simulink model "Simplified_UAV_Task3"  (R2024b)
settings: Solver=VariableStepAuto  StartTime=0  StopTime=3000  FixedStep=1e-4  RelTol=1e-5  AbsTol=1e-5
values from neighbouring files (symbols this model uses):
  adaptiveActivation = 1    [Simplified_UAV_Task3_main.m]    (also in newUAV_Task3_main.m)
  B_p = 1/UAV.m    [Simplified_UAV_Task3_main.m]    (also in newUAV_Task3_main.m)
  Gamma_a = 1*[1 1 1 1]'    [Simplified_UAV_Task3_main.m]    (also in newUAV_Task3_main.m = 2*[1 1 1 1]')
  gravityInAdaptiveController = 1    [Simplified_UAV_Task3_main.m]    (also in newUAV_Task3_main.m)
  L = 10    [Simplified_UAV_Task3_main.m]    (also in newUAV_Task3_main.m)
  lambda = 0.89    [Simplified_UAV_Task3_main.m]    (also in newUAV_Task3_main.m)
  lambda_0 = 1    [Simplified_UAV_Task3_main.m]    (also in newUAV_Task3_main.m)
  p_0 = [0; 0; 0]    [Simplified_UAV_Task3_main.m]    (also in newUAV_Task3_main.m)
  PO = 1    [Simplified_UAV_Task3_main.m]    (also in newUAV_Task3_main.m)
  scenario = 2    [Simplified_UAV_Task3_main.m]    (also in newUAV_Task3_main.m)
  theta_0 = [0.07;0.07;0.1]    [Simplified_UAV_Task3_main.m]    (also in newUAV_Task3_main.m)
  vb_0 = [0; 0; 0]    [Simplified_UAV_Task3_main.m]    (also in newUAV_Task3_main.m)
undefined symbols (not defined in the file or in its folder): ctrl, epsilon_PO, g, Gamma_a_scalar, par, projection_operator, targetParams, theta_M, UAV, v_0
libraries: matrix_library x12, slpidlib x12, spsRMSLib x1, uavutilslib x1
(part 3 of 3)

== system Simplified_UAV_Task3/Position Controller/ADAPTIVE CONTROLLER/Subsystem1 ==
  u_b : Inport
  lambda : Inport  Port=2
  xp : Inport  Port=3
  thetap_hat : Inport  Port=4
  Constant : Constant
  Create Diagonal Matrix : matrix_library/Create Diagonal Matrix
  Gain2 : Gain  Gain=-1
  MATLAB Function1 : MATLAB Function  TreatAsAtomicUnit=on
  Matrix Multiply : Product
  Matrix Multiply1 : Product  Multiplication=Matrix(*)
  Matrix Multiply2 : Product
  Sum : Sum  Inputs=+-
  Sum1 : Sum  Inputs=+-
  Sum2 : Sum
  u_a : Outport
  u : Outport  Port=2
  wires:
  lambda/1 -> MATLAB Function1/1(lambda)
  MATLAB Function1/1(Lambda_hat_inv) -> Matrix Multiply2/1, Sum/1
  Constant/1 -> Sum/2
  Sum/1 -> Matrix Multiply/1
  u_b/1 -> Sum2/2, Matrix Multiply/2
  Matrix Multiply/1 -> Sum1/1
  xp/1 -> Create Diagonal Matrix/1
  thetap_hat/1 -> Matrix Multiply1/2
  Sum1/1 -> Sum2/1, u_a/1
  Sum2/1 -> u/1
  Create Diagonal Matrix/1 -> Gain2/1
  Gain2/1 -> Matrix Multiply1/1
  Matrix Multiply1/1 -> Matrix Multiply2/2
  Matrix Multiply2/1 -> Sum1/2

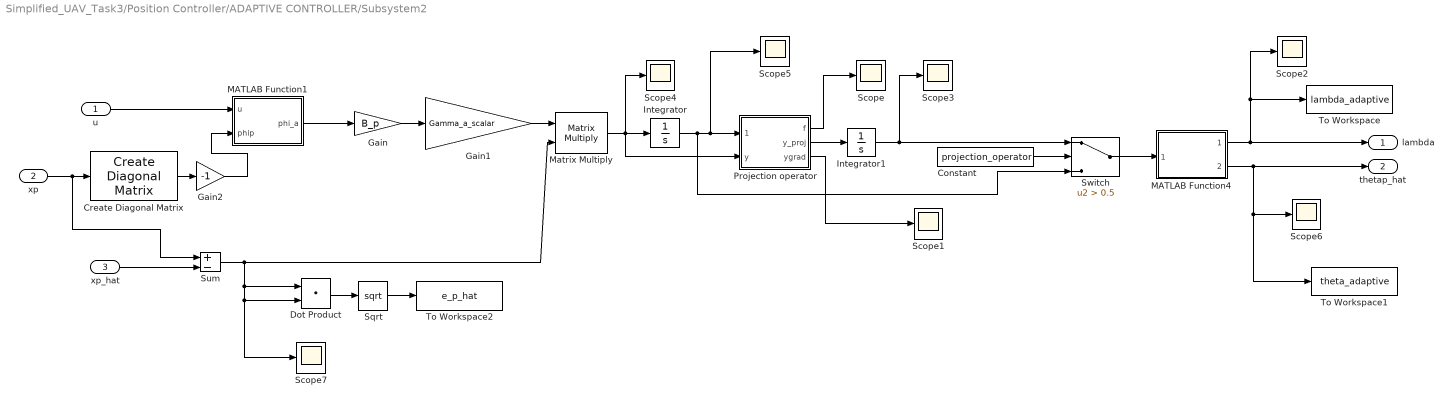
== system Simplified_UAV_Task3/Position Controller/ADAPTIVE CONTROLLER/Subsystem2 ==
  u : Inport
  xp : Inport  Port=2
  xp_hat : Inport  Port=3
  Constant : Constant  Value=projection_operator
  Create Diagonal Matrix : matrix_library/Create Diagonal Matrix
  Dot Product : DotProduct  OutDataTypeStr=Inherit: Inherit via internal rule
  Gain : Gain  Gain=B_p
  Gain1 : Gain  Gain=Gamma_a_scalar
  Gain2 : Gain  Gain=-1
  Integrator : Integrator  InitialCondition=[lambda_0; theta_0]
  Integrator1 : Integrator  InitialCondition=[lambda_0; theta_0]
  MATLAB Function1 : MATLAB Function  TreatAsAtomicUnit=on
  MATLAB Function4 : MATLAB Function  TreatAsAtomicUnit=on
  Matrix Multiply : Product  Multiplication=Matrix(*)
  Projection operator : MATLAB Function  TreatAsAtomicUnit=on
  Scope{,1..7} (8 alike) : Scope
  Sqrt : Sqrt
  Sum : Sum  Inputs=+-
  Switch : Switch  Criteria=u2 > Threshold  Threshold=0.5  SaturateOnIntegerOverflow=off  InputSameDT=off
  To Workspace : ToWorkspace  VariableName=lambda_adaptive  SaveFormat=Timeseries  SampleTime=-1
  To Workspace1 : ToWorkspace  VariableName=theta_adaptive  SaveFormat=Timeseries  SampleTime=-1
  To Workspace2 : ToWorkspace  VariableName=e_p_hat  SaveFormat=Timeseries  SampleTime=-1
  lambda : Outport
  thetap_hat : Outport  Port=2
  wires:
  u/1 -> MATLAB Function1/1(u)
  xp_hat/1 -> Sum/2
  MATLAB Function1/1(phi_a) -> Gain/1
  Gain/1 -> Gain1/1
  Gain1/1 -> Matrix Multiply/1
  Matrix Multiply/1 -> Projection operator/2(y), Scope4/1, Integrator/1
  Integrator/1 -> Switch/3, Scope5/1, Projection operator/1(theta_a_hat)
  Projection operator/3(ygrad) -> Scope1/1
  Projection operator/1(f) -> Scope/1
  MATLAB Function4/2(thetap_hat) -> To Workspace1/1, Scope6/1, thetap_hat/1
  Integrator1/1 -> Switch/1, Scope3/1
  Projection operator/2(y_proj) -> Integrator1/1
  xp/1 -> Create Diagonal Matrix/1, Sum/1
  Switch/1 -> MATLAB Function4/1(theta_a)
  Constant/1 -> Switch/2
  Create Diagonal Matrix/1 -> Gain2/1
  Gain2/1 -> MATLAB Function1/2(phip)
  Sqrt/1 -> To Workspace2/1
  Sum/1 -> Scope7/1, Dot Product/2, Dot Product/1, Matrix Multiply/2
  Dot Product/1 -> Sqrt/1
  MATLAB Function4/1(lambda) -> lambda/1, To Workspace/1, Scope2/1

== system Simplified_UAV_Task3/Position Controller/Adaptive Augmentation/Predictor (x_p_hat) dynamics ==
  Lambda_hat : Inport
  u : Inport  Port=2
  phi_p : Inport  Port=3
  theta_p_hat : Inport  Port=4
  x_p : Inport  Port=5
  Add : Sum
  Constant : Constant  Value=g*e3
  Gain : Gain  Gain=B_p  Multiplication=Matrix(K*u)
  Gain1 : Gain  Gain=L
  Gain2 : Gain  Gain=gravityInAdaptiveController
  Gain3 : Gain
  Integrator : Integrator  InitialCondition=v_0
  Matrix Multiply : Product
  Matrix Multiply1 : Product  Multiplication=Matrix(*)
  Reshape : Reshape  OutputDimensionality=Column vector (2-D)
  Reshape1 : Reshape  OutputDimensionality=Column vector (2-D)
  Reshape2 : Reshape  OutputDimensionality=Column vector (2-D)
  Scope : Scope
  Scope1 : Scope
  Sum : Sum  Inputs=+++
  Sum1 : Sum  Inputs=-+|
  Transpose : Math  Operator=transpose
  x_p_hat : Outport
  wires:
  Lambda_hat/1 -> Matrix Multiply/1
  Matrix Multiply/1 -> Add/1
  phi_p/1 -> Transpose/1
  theta_p_hat/1 -> Matrix Multiply1/2
  Matrix Multiply1/1 -> Add/2
  Add/1 -> Gain/1
  Gain/1 -> Reshape1/1
  Gain1/1 -> Reshape/1
  x_p/1 -> Scope1/1, Sum1/2
  Sum1/1 -> Gain1/1
  Integrator/1 -> Scope/1, Sum1/1, x_p_hat/1
  Sum/1 -> Integrator/1
  Reshape/1 -> Sum/1
  Reshape1/1 -> Sum/2
  Reshape2/1 -> Sum/3
  Constant/1 -> Gain2/1
  Transpose/1 -> Matrix Multiply1/1
  u/1 -> Matrix Multiply/2
  Gain2/1 -> Gain3/1
  Gain3/1 -> Reshape2/1

== system Simplified_UAV_Task3/Position Controller/Adaptive Augmentation/Subsystem ==
  Lambda_hat : Inport
  u_b : Inport  Port=2
  phi_p : Inport  Port=3
  theta_p_hat : Inport  Port=4
  Constant : Constant  Value=eye(3,3)
  Gain : Gain  Commented=through  Gain=-1
  Gain1 : Gain
  Inverse : MATLAB Function  TreatAsAtomicUnit=on
  Product : Product  Multiplication=Matrix(*)
  Product1 : Product  Inputs=3  Multiplication=Matrix(*)
  Subtract : Sum  Inputs=-+
  Subtract1 : Sum  Inputs=+-
  Transpose : Math  Operator=transpose
  u_a : Outport
  wires:
  Lambda_hat/1 -> Inverse/1(u)
  Inverse/1(y) -> Product1/1, Subtract/2
  Constant/1 -> Subtract/1
  Subtract/1 -> Product/1
  u_b/1 -> Product/2
  Product/1 -> Gain1/1
  Subtract1/1 -> u_a/1
  phi_p/1 -> Transpose/1
  Transpose/1 -> Gain/1
  theta_p_hat/1 -> Product1/3
  Product1/1 -> Subtract1/2
  Gain/1 -> Product1/2
  Gain1/1 -> Subtract1/1

== system Simplified_UAV_Task3/Position Controller/Adaptive Augmentation/phi_a ==
  u : Inport
  phi_p : Inport  Port=2
  Matrix Concatenate : Concatenate  Mode=Multidimensional array
  Scope : Scope
  Transpose : Math  Operator=transpose
  phi_a : Outport
  wires:
  Matrix Concatenate/1 -> Scope/1, phi_a/1
  u/1 -> Transpose/1
  phi_p/1 -> Matrix Concatenate/2
  Transpose/1 -> Matrix Concatenate/1

== system Simplified_UAV_Task3/Position Controller/Adaptive Augmentation/phi_p ==
  x_p : Inport
  Create Diagonal Matrix : matrix_library/Create Diagonal Matrix
  Gain : Gain  Gain=-1
  phi_p : Outport
  wires:
  x_p/1 -> Gain/1
  Gain/1 -> Create Diagonal Matrix/1
  Create Diagonal Matrix/1 -> phi_p/1

== system Simplified_UAV_Task3/Position Controller/Adaptive Augmentation/theta_a_hat dynamics ==
  Gamma_a : Inport
  phi_a : Inport  Port=2
  B_p : Inport  Port=3
  x_p : Inport  Port=4
  x_p_hat : Inport  Port=5
  Constant1 : Constant  Value=PO
  Dot Product : DotProduct  OutDataTypeStr=Inherit: Inherit via internal rule
  Integrator : Integrator  InitialCondition=[lambda_0; theta_0]
  Matrix Multiply1 : Product
  Matrix Multiply2 : Product  Multiplication=Matrix(*)
  Matrix Multiply3 : Product
  Projection operator : Subsystem
  Scope{,1..4} (5 alike) : Scope
  Sqrt : Sqrt
  Subtract : Sum  Inputs=+-
  Switch : Switch  Criteria=u2 > Threshold  SaturateOnIntegerOverflow=off  InputSameDT=off
  To Workspace : ToWorkspace  VariableName=e_p_hat  SaveFormat=Timeseries  SampleTime=-1
  Transpose : Math  Operator=transpose
  Transpose1 : Math  Commented=through  Operator=transpose
  theta_a_hat : Outport
  wires:
  x_p_hat/1 -> Subtract/2
  B_p/1 -> Transpose/1
  Subtract/1 -> Scope4/1, Dot Product/2, Dot Product/1, Matrix Multiply1/2
  Transpose/1 -> Matrix Multiply1/1
  phi_a/1 -> Transpose1/1
  Matrix Multiply1/1 -> Scope3/1, Matrix Multiply2/2
  Gamma_a/1 -> Matrix Multiply3/1
  Matrix Multiply2/1 -> Matrix Multiply3/2
  Matrix Multiply3/1 -> Projection operator/1(theta_dot), Scope2/1, Integrator/1
  x_p/1 -> Subtract/1
  Constant1/1 -> Switch/2, Projection operator/Enable
  Integrator/1 -> Scope1/1, Switch/3
  Switch/1 -> theta_a_hat/1
  Projection operator/1(theta) -> Scope/1, Switch/1
  Dot Product/1 -> Sqrt/1
  Sqrt/1 -> To Workspace/1
  Transpose1/1 -> Matrix Multiply2/1

== system Simplified_UAV_Task3/Position Controller/Adaptive Augmentation to delete/Predictor (x_p_hat) dynamics ==
  Lambda_hat : Inport
  u : Inport  Port=2
  phi_p : Inport  Port=3
  theta_p_hat : Inport  Port=4
  x_p : Inport  Port=5
  Add : Sum
  Constant : Constant  Value=g*e3
  Gain : Gain  Gain=B_p  Multiplication=Matrix(K*u)
  Gain1 : Gain  Gain=L
  Integrator : Integrator  InitialCondition=v_0
  Matrix Multiply : Product
  Matrix Multiply1 : Product  Multiplication=Matrix(*)
  Reshape : Reshape  OutputDimensionality=Column vector (2-D)
  Reshape1 : Reshape  OutputDimensionality=Column vector (2-D)
  Reshape2 : Reshape  OutputDimensionality=Column vector (2-D)
  Scope : Scope
  Sum : Sum  Inputs=+++
  Sum1 : Sum  Inputs=-+|
  Transpose : Math  Operator=transpose
  x_p_hat : Outport
  wires:
  Lambda_hat/1 -> Matrix Multiply/1
  u/1 -> Matrix Multiply/2
  Matrix Multiply/1 -> Add/1
  phi_p/1 -> Transpose/1
  theta_p_hat/1 -> Matrix Multiply1/2
  Matrix Multiply1/1 -> Add/2
  Add/1 -> Gain/1
  Gain/1 -> Reshape1/1
  Gain1/1 -> Reshape/1
  x_p/1 -> Sum1/2
  Sum1/1 -> Gain1/1
  Integrator/1 -> Scope/1, Sum1/1, x_p_hat/1
  Sum/1 -> Integrator/1
  Reshape/1 -> Sum/1
  Reshape1/1 -> Sum/2
  Reshape2/1 -> Sum/3
  Constant/1 -> Reshape2/1
  Transpose/1 -> Matrix Multiply1/1

== system Simplified_UAV_Task3/Position Controller/Adaptive Augmentation to delete/Subsystem ==
  Lambda_hat : Inport
  u_b : Inport  Port=2
  phi_p : Inport  Port=3
  theta_p_hat : Inport  Port=4
  Constant : Constant  Value=eye(3,3)
  Gain : Gain  Commented=through  Gain=-1
  Gain1 : Gain
  Inverse : MATLAB Function  TreatAsAtomicUnit=on
  Product : Product  Multiplication=Matrix(*)
  Product1 : Product  Inputs=3  Multiplication=Matrix(*)
  Subtract : Sum  Inputs=-+
  Subtract1 : Sum  Inputs=+-
  Transpose : Math  Operator=transpose
  u_a : Outport
  wires:
  Lambda_hat/1 -> Inverse/1(u)
  Inverse/1(y) -> Product1/1, Subtract/2
  Constant/1 -> Subtract/1
  Subtract/1 -> Product/1
  u_b/1 -> Product/2
  Product/1 -> Gain1/1
  Subtract1/1 -> u_a/1
  phi_p/1 -> Transpose/1
  Transpose/1 -> Gain/1
  theta_p_hat/1 -> Product1/3
  Product1/1 -> Subtract1/2
  Gain/1 -> Product1/2
  Gain1/1 -> Subtract1/1

== system Simplified_UAV_Task3/Position Controller/Adaptive Augmentation to delete/phi_a ==
  u : Inport
  phi_p : Inport  Port=2
  Matrix Concatenate : Concatenate  Mode=Multidimensional array
  Scope : Scope
  Transpose : Math  Operator=transpose
  phi_a : Outport
  wires:
  Matrix Concatenate/1 -> Scope/1, phi_a/1
  u/1 -> Transpose/1
  phi_p/1 -> Matrix Concatenate/2
  Transpose/1 -> Matrix Concatenate/1

== system Simplified_UAV_Task3/Position Controller/Adaptive Augmentation to delete/phi_p ==
  x_p : Inport
  Create Diagonal Matrix : matrix_library/Create Diagonal Matrix
  Gain : Gain  Gain=-1
  phi_p : Outport
  wires:
  x_p/1 -> Gain/1
  Gain/1 -> Create Diagonal Matrix/1
  Create Diagonal Matrix/1 -> phi_p/1

== system Simplified_UAV_Task3/Position Controller/Adaptive Augmentation to delete/theta_a_hat dynamics ==
  Gamma_a : Inport
  phi_a : Inport  Port=2
  B_p : Inport  Port=3
  x_p : Inport  Port=4
  x_p_hat : Inport  Port=5
  Constant1 : Constant  Value=PO
  Dot Product : DotProduct  OutDataTypeStr=Inherit: Inherit via internal rule
  Integrator : Integrator  InitialCondition=[lambda_0; theta_0]
  Matrix Multiply1 : Product
  Matrix Multiply2 : Product  Multiplication=Matrix(*)
  Matrix Multiply3 : Product
  Projection operator : Subsystem  Commented=on
  Scope{,1..4} (5 alike) : Scope
  Sqrt : Sqrt
  Subtract : Sum  Inputs=+-
  Switch : Switch  Criteria=u2 > Threshold  SaturateOnIntegerOverflow=off  InputSameDT=off
  To Workspace : ToWorkspace  VariableName=e_p_hat  SaveFormat=Timeseries  SampleTime=-1
  Transpose : Math  Operator=transpose
  Transpose1 : Math  Commented=through  Operator=transpose
  theta_a_hat : Outport
  wires:
  x_p_hat/1 -> Subtract/2
  B_p/1 -> Transpose/1
  Subtract/1 -> Matrix Multiply1/2, Scope4/1, Dot Product/2, Dot Product/1
  Transpose/1 -> Matrix Multiply1/1
  phi_a/1 -> Transpose1/1
  Matrix Multiply1/1 -> Scope3/1, Matrix Multiply2/2
  Gamma_a/1 -> Matrix Multiply3/1
  Matrix Multiply2/1 -> Matrix Multiply3/2
  Matrix Multiply3/1 -> Projection operator/1(theta_dot), Scope2/1, Integrator/1
  x_p/1 -> Subtract/1
  Constant1/1 -> Switch/2, Projection operator/Enable
  Integrator/1 -> Scope1/1, Switch/3
  Switch/1 -> theta_a_hat/1
  Projection operator/1(theta) -> Scope/1, Switch/1
  Dot Product/1 -> Sqrt/1
  Sqrt/1 -> To Workspace/1
  Transpose1/1 -> Matrix Multiply2/1

== system Simplified_UAV_Task3/Position Controller/position/Subsystem ==
  e_p : Inport
  Action Port : ActionPort
  Dot Product : DotProduct  OutDataTypeStr=Inherit: Inherit via internal rule
  Sqrt : Sqrt
  Sum of Elements : Sum  Inputs=+
  To Workspace : ToWorkspace  VariableName=posRMS  SaveFormat=Timeseries  SampleTime=-1
  wires:
  e_p/1 -> Dot Product/2, Dot Product/1
  Dot Product/1 -> Sum of Elements/1
  Sum of Elements/1 -> Sqrt/1
  Sqrt/1 -> To Workspace/1

== system Simplified_UAV_Task3/Position Controller/velocity/Subsystem ==
  e_p : Inport
  Action Port : ActionPort
  Dot Product : DotProduct  OutDataTypeStr=Inherit: Inherit via internal rule
  Sqrt : Sqrt
  Sum of Elements : Sum  Inputs=+
  To Workspace : ToWorkspace  VariableName=velRMS  SaveFormat=Timeseries  SampleTime=-1
  wires:
  e_p/1 -> Dot Product/2, Dot Product/1
  Dot Product/1 -> Sum of Elements/1
  Sum of Elements/1 -> Sqrt/1
  Sqrt/1 -> To Workspace/1

== system Simplified_UAV_Task3/Classic Position Controller/Adaptive Augmentation/theta_a_hat dynamics/Projection operator ==
  theta_dot : Inport
  Enable : EnablePort
  Constant : Constant  Value=lambda_0
  Constant3 : Constant  Value=theta_0(1)
  Constant4 : Constant  Value=theta_0(2)
  Constant5 : Constant  Value=theta_0(3)
  Demux : Demux
  Integrator{1,4..6} (4 alike) : Integrator
  MATLAB Function : MATLAB Function  TreatAsAtomicUnit=on
  MATLAB Function3 : MATLAB Function  TreatAsAtomicUnit=on
  MATLAB Function4 : MATLAB Function  TreatAsAtomicUnit=on
  MATLAB Function5 : MATLAB Function  TreatAsAtomicUnit=on
  Mux : Mux
  Sum{,3..5} (4 alike) : Sum  Inputs=|++
  theta : Outport
  wires:
  MATLAB Function/1(y_proj) -> Integrator1/1
  Sum/1 -> MATLAB Function/1(theta), Mux/1
  Integrator1/1 -> Sum/1
  Constant/1 -> Sum/2
  Demux/1 -> MATLAB Function/2(theta_dot)
  theta_dot/1 -> Demux/1
  Constant3/1 -> Sum3/2
  MATLAB Function3/1(y_proj) -> Integrator4/1
  Sum3/1 -> Mux/2, MATLAB Function3/1(theta)
  Integrator4/1 -> Sum3/1
  Demux/2 -> MATLAB Function3/2(theta_dot)
  Constant4/1 -> Sum4/2
  MATLAB Function4/1(y_proj) -> Integrator5/1
  Sum4/1 -> Mux/3, MATLAB Function4/1(theta)
  Integrator5/1 -> Sum4/1
  Demux/3 -> MATLAB Function4/2(theta_dot)
  Constant5/1 -> Sum5/2
  MATLAB Function5/1(y_proj) -> Integrator6/1
  Sum5/1 -> MATLAB Function5/1(theta), Mux/4
  Integrator6/1 -> Sum5/1
  Demux/4 -> MATLAB Function5/2(theta_dot)
  Mux/1 -> theta/1

== system Simplified_UAV_Task3/Position Controller/Adaptive Augmentation/theta_a_hat dynamics/Projection operator ==
  theta_dot : Inport
  Enable : EnablePort
  Constant : Constant  Value=lambda_0
  Constant3 : Constant  Value=theta_0(1)
  Constant4 : Constant  Value=theta_0(2)
  Constant5 : Constant  Value=theta_0(3)
  Demux : Demux
  Integrator{1,4..6} (4 alike) : Integrator
  MATLAB Function : MATLAB Function  TreatAsAtomicUnit=on
  MATLAB Function3 : MATLAB Function  TreatAsAtomicUnit=on
  MATLAB Function4 : MATLAB Function  TreatAsAtomicUnit=on
  MATLAB Function5 : MATLAB Function  TreatAsAtomicUnit=on
  Mux : Mux
  Sum{,3..5} (4 alike) : Sum  Inputs=|++
  theta : Outport
  wires:
  MATLAB Function/1(y_proj) -> Integrator1/1
  Sum/1 -> MATLAB Function/1(theta), Mux/1
  Integrator1/1 -> Sum/1
  Constant/1 -> Sum/2
  Demux/1 -> MATLAB Function/2(theta_dot)
  theta_dot/1 -> Demux/1
  Constant3/1 -> Sum3/2
  MATLAB Function3/1(y_proj) -> Integrator4/1
  Sum3/1 -> Mux/2, MATLAB Function3/1(theta)
  Integrator4/1 -> Sum3/1
  Demux/2 -> MATLAB Function3/2(theta_dot)
  Constant4/1 -> Sum4/2
  MATLAB Function4/1(y_proj) -> Integrator5/1
  Sum4/1 -> Mux/3, MATLAB Function4/1(theta)
  Integrator5/1 -> Sum4/1
  Demux/3 -> MATLAB Function4/2(theta_dot)
  Constant5/1 -> Sum5/2
  MATLAB Function5/1(y_proj) -> Integrator6/1
  Sum5/1 -> MATLAB Function5/1(theta), Mux/4
  Integrator6/1 -> Sum5/1
  Demux/4 -> MATLAB Function5/2(theta_dot)
  Mux/1 -> theta/1

== system Simplified_UAV_Task3/Position Controller/Adaptive Augmentation to delete/theta_a_hat dynamics/Projection operator ==
  theta_dot : Inport
  Enable : EnablePort
  Constant : Constant  Value=lambda_0
  Constant3 : Constant  Value=theta_0(1)
  Constant4 : Constant  Value=theta_0(2)
  Constant5 : Constant  Value=theta_0(3)
  Demux : Demux
  Integrator{1,4..6} (4 alike) : Integrator
  MATLAB Function : MATLAB Function  TreatAsAtomicUnit=on
  MATLAB Function3 : MATLAB Function  TreatAsAtomicUnit=on
  MATLAB Function4 : MATLAB Function  TreatAsAtomicUnit=on
  MATLAB Function5 : MATLAB Function  TreatAsAtomicUnit=on
  Mux : Mux
  Sum{,3..5} (4 alike) : Sum  Inputs=|++
  theta : Outport
  wires:
  MATLAB Function/1(y_proj) -> Integrator1/1
  Sum/1 -> MATLAB Function/1(theta), Mux/1
  Integrator1/1 -> Sum/1
  Constant/1 -> Sum/2
  Demux/1 -> MATLAB Function/2(theta_dot)
  theta_dot/1 -> Demux/1
  Constant3/1 -> Sum3/2
  MATLAB Function3/1(y_proj) -> Integrator4/1
  Sum3/1 -> Mux/2, MATLAB Function3/1(theta)
  Integrator4/1 -> Sum3/1
  Demux/2 -> MATLAB Function3/2(theta_dot)
  Constant4/1 -> Sum4/2
  MATLAB Function4/1(y_proj) -> Integrator5/1
  Sum4/1 -> Mux/3, MATLAB Function4/1(theta)
  Integrator5/1 -> Sum4/1
  Demux/3 -> MATLAB Function4/2(theta_dot)
  Constant5/1 -> Sum5/2
  MATLAB Function5/1(y_proj) -> Integrator6/1
  Sum5/1 -> MATLAB Function5/1(theta), Mux/4
  Integrator6/1 -> Sum5/1
  Demux/4 -> MATLAB Function5/2(theta_dot)
  Mux/1 -> theta/1

== matlab function Simplified_UAV_Task3/Adaptive Augmentation 6 parameters/theta_a_hat dynamics/Projection operator/MATLAB Function5 ==
  data: theta input; y_proj output; theta_dot input; par parameter
function y_proj = proj(theta,theta_dot,par)

% I could get rid of the center by not feeding it to the function

Gamma = par.Gamma(6);
eps_proj = par.eps_proj;
theta_M = par.theta_M(6);
center = par.center(6);
theta = theta - center;

f = 1/(eps_proj*theta_M^2)*((1+eps_proj)*(theta')*theta-theta_M^2);
grad_f = 2/(eps_proj*theta_M^2)*(1+eps_proj)*theta;

if f>0 && all(theta_dot'*Gamma*grad_f>0)
    y_proj = Gamma*theta_dot - f*Gamma*(grad_f)*grad_f'/(grad_f'*Gamma*grad_f)*Gamma*theta_dot;
else
    y_proj = Gamma*theta_dot;
end

== matlab function Simplified_UAV_Task3/Main Trajectory Generation ==
  data: v_b_dot output size=[3,1]; v_b output size=[3,1]; p output size=[3,1]; time input; targetParams parameter; scenario parameter
function [v_b_dot, v_b, p]   = fcn(time, targetParams, scenario)

activation = 0;
rateOfClimb = 0.3*activation*0;

if scenario == 1
    v_b_dot = targetParams.v_b_dot;
    v_b = targetParams.v_b;
    p = targetParams.p;
else
    angle = 2*pi/60*time;
    p = 3*[sin(angle); cos(angle); -2/3-rateOfClimb*time/3+1/3*(cos(angle)+sin(angle))*activation];
    v_b = pi/10*[cos(angle); -sin(angle); -rateOfClimb/pi*10-1/pi*10*(sin(angle)-cos(angle))*activation];
    v_b_dot = ((pi/10)^2)/3*[-sin(angle); -cos(angle); -1/(((pi/10)^2)/3)*(cos(angle)-sin(angle))*activation];
end

== matlab function Simplified_UAV_Task3/Position Controller/Adaptive Augmentation to delete/Subsystem/Inverse ==
  data: u input; y output
function y = fcn(u)

Lambda = diag([u;u;u]);
y = inv(Lambda);

== matlab function Simplified_UAV_Task3/Position Controller/Adaptive Augmentation to delete/theta_a_hat dynamics/Projection operator/MATLAB Function ==
  data: theta input; y_proj output; theta_dot input; par parameter
function y_proj = proj(theta,theta_dot,par)

% I could get rid of the center by not feeding it to the function

Gamma = par.Gamma(1);
eps_proj = par.eps_proj;
theta_M = par.theta_M(1);
center = par.center(1);
theta = theta - center;

f = 1/(eps_proj*theta_M^2)*((1+eps_proj)*(theta')*theta-theta_M^2);
grad_f = 2/(eps_proj*theta_M^2)*(1+eps_proj)*theta;

if f>0 && all(theta_dot'*Gamma*grad_f>0)
    y_proj = Gamma*theta_dot - f*Gamma*(grad_f)*grad_f'/(grad_f'*Gamma*grad_f)*Gamma*theta_dot;
else
    y_proj = Gamma*theta_dot;
end

== matlab function Simplified_UAV_Task3/Position Controller/Adaptive Augmentation to delete/theta_a_hat dynamics/Projection operator/MATLAB Function3 ==
  data: theta input; y_proj output; theta_dot input; par parameter
function y_proj = proj(theta,theta_dot,par)

% I could get rid of the center by not feeding it to the function

Gamma = par.Gamma(4);
eps_proj = par.eps_proj;
theta_M = par.theta_M(4);
center = par.center(4);
theta = theta - center;

f = 1/(eps_proj*theta_M^2)*((1+eps_proj)*(theta')*theta-theta_M^2);
grad_f = 2/(eps_proj*theta_M^2)*(1+eps_proj)*theta;

if f>0 && all(theta_dot'*Gamma*grad_f>0)
    y_proj = Gamma*theta_dot - f*Gamma*(grad_f)*grad_f'/(grad_f'*Gamma*grad_f)*Gamma*theta_dot;
else
    y_proj = Gamma*theta_dot;
end

== matlab function Simplified_UAV_Task3/ADAPTIVE CONTROLLER/Subsystem/MATLAB Function1 ==
  data: lambda input; Lambda_hat output
function Lambda_hat = fcn(lambda)

Lambda_hat = [lambda 0 0; 0 lambda 0; 0 0 lambda];

== matlab function Simplified_UAV_Task3/Position Controller/Adaptive Augmentation to delete/theta_a_hat dynamics/Projection operator/MATLAB Function4 ==
  data: theta input; y_proj output; theta_dot input; par parameter
function y_proj = proj(theta,theta_dot,par)

% I could get rid of the center by not feeding it to the function

Gamma = par.Gamma(5);
eps_proj = par.eps_proj;
theta_M = par.theta_M(5);
center = par.center(5);
theta = theta - center;

f = 1/(eps_proj*theta_M^2)*((1+eps_proj)*(theta')*theta-theta_M^2);
grad_f = 2/(eps_proj*theta_M^2)*(1+eps_proj)*theta;

if f>0 && all(theta_dot'*Gamma*grad_f>0)
    y_proj = Gamma*theta_dot - f*Gamma*(grad_f)*grad_f'/(grad_f'*Gamma*grad_f)*Gamma*theta_dot;
else
    y_proj = Gamma*theta_dot;
end

== matlab function Simplified_UAV_Task3/Position Controller/ADAPTIVE CONTROLLER/Subsystem/MATLAB Function1 ==
  data: lambda input; Lambda_hat output
function Lambda_hat = fcn(lambda)

Lambda_hat = [lambda 0 0; 0 lambda 0; 0 0 lambda];

== matlab function Simplified_UAV_Task3/Position Controller/Adaptive Augmentation to delete/theta_a_hat dynamics/Projection operator/MATLAB Function5 ==
  data: theta input; y_proj output; theta_dot input; par parameter
function y_proj = proj(theta,theta_dot,par)

% I could get rid of the center by not feeding it to the function

Gamma = par.Gamma(4);
eps_proj = par.eps_proj;
theta_M = par.theta_M(4);
center = par.center(4);
theta = theta - center;

f = 1/(eps_proj*theta_M^2)*((1+eps_proj)*(theta')*theta-theta_M^2);
grad_f = 2/(eps_proj*theta_M^2)*(1+eps_proj)*theta;

if f>0 && all(theta_dot'*Gamma*grad_f>0)
    y_proj = Gamma*theta_dot - f*Gamma*(grad_f)*grad_f'/(grad_f'*Gamma*grad_f)*Gamma*theta_dot;
else
    y_proj = Gamma*theta_dot;
end

== matlab function Simplified_UAV_Task3/Adaptive Augmentation/theta_a_hat dynamics/Projection operator/MATLAB Function ==
  data: theta input; y_proj output; theta_dot input; par parameter
function y_proj = proj(theta,theta_dot,par)

% I could get rid of the center by not feeding it to the function

Gamma = par.Gamma(1);
eps_proj = par.eps_proj;
theta_M = par.theta_M(1);
center = par.center(1);
theta = theta - center;

f = 1/(eps_proj*theta_M^2)*((1+eps_proj)*(theta')*theta-theta_M^2);
grad_f = 2/(eps_proj*theta_M^2)*(1+eps_proj)*theta;

if f>0 && all(theta_dot'*Gamma*grad_f>0)
    y_proj = Gamma*theta_dot - f*Gamma*(grad_f)*grad_f'/(grad_f'*Gamma*grad_f)*Gamma*theta_dot;
else
    y_proj = Gamma*theta_dot;
end

== matlab function Simplified_UAV_Task3/ADAPTIVE CONTROLLER/Subsystem2/MATLAB Function1 ==
  data: u input; phi_a output; phip input
function phi_a = fcn(u, phip)

phi_a = [u(1,1), u(2,1), u(3,1);
    phip(1,1), phip(1,2), phip(1,3);
    phip(2,1), phip(2,2), phip(2,3);
    phip(3,1), phip(3,2), phip(3,3)];

== matlab function Simplified_UAV_Task3/ADAPTIVE CONTROLLER/Subsystem2/MATLAB Function4 ==
  data: theta_a input; lambda output; thetap_hat output
function [lambda, thetap_hat] = fcn(theta_a)

lambda = theta_a(1);
thetap_hat = [theta_a(2) theta_a(3) theta_a(4)]';

== matlab function Simplified_UAV_Task3/ADAPTIVE CONTROLLER/Subsystem2/Projection operator ==
  data: f output; theta_a_hat input; y_proj output; y input; epsilon_PO parameter; theta_M parameter; ygrad output
function [f, y_proj, ygrad] = fcn(theta_a_hat, y, epsilon_PO, theta_M)

% 1
f_1 = ((1 + epsilon_PO(1))*theta_a_hat(1)^2 - theta_M(1)^2)/(epsilon_PO(1)*theta_M(1)^2);
grad_f_1 = 2*(1 + epsilon_PO(1))*theta_a_hat(1)/(epsilon_PO(1)*theta_M(1)^2);

if f_1>0 && y(1)*grad_f_1>0
    y_proj_1 = y(1) - f_1*(grad_f_1^2)/grad_f_1^2*y(1);
else
    y_proj_1 = y(1);
end

% 2
f_2 = ((2 + epsilon_PO(2))*theta_a_hat(2)^2 - theta_M(2)^2)/(epsilon_PO(2)*theta_M(2)^2);
grad_f_2 = 2*(2 + epsilon_PO(2))*theta_a_hat(2)/(epsilon_PO(2)*theta_M(2)^2);

if f_2>0 && y(2)*grad_f_2>0
    y_proj_2 = y(2) - f_2*(grad_f_2^2)/grad_f_2^2*y(2);
else
    y_proj_2 = y(2);
end

% 3
f_3 = ((3 + epsilon_PO(3))*theta_a_hat(3)^2 - theta_M(3)^2)/(epsilon_PO(3)*theta_M(3)^2);
grad_f_3 = 2*(3 + epsilon_PO(3))*theta_a_hat(3)/(epsilon_PO(3)*theta_M(3)^2);

if f_3>0 && y(3)*grad_f_3>0
    y_proj_3 = y(3) - f_3*(grad_f_3^2)/grad_f_3^2*y(3);
else
    y_proj_3 = y(3);
end

% 4
f_4 = ((4 + epsilon_PO(4))*theta_a_hat(4)^2 - theta_M(4)^2)/(epsilon_PO(4)*theta_M(4)^2);
grad_f_4 = 2*(4 + epsilon_PO(4))*theta_a_hat(4)/(epsilon_PO(4)*theta_M(4)^2);

if f_4>0 && y(4)*grad_f_4>0
    y_proj_4 = y(4) - f_4*(grad_f_4^2)/grad_f_4^2*y(4);
else
    y_proj_4 = y(4);
end

f = [f_1, f_2, f_3, f_4]';
y_proj = [y_proj_1, y_proj_2, y_proj_3, y_proj_4]';
grad_f = [grad_f_1, grad_f_2, grad_f_3, grad_f_4]';
ygrad = [y(1)*grad_f_1, y(2)*grad_f_2, y(3)*grad_f_3, y(4)*grad_f_4];

== matlab function Simplified_UAV_Task3/Position Controller/ADAPTIVE CONTROLLER/Subsystem1/MATLAB Function1 ==
  data: lambda input; Lambda_hat_inv output
function Lambda_hat_inv = fcn(lambda)

%lambda_hat = [lambda 0 0; 0 lambda 0; 0 0 lambda];
Lambda_hat_inv = inv(lambda);

== matlab function Simplified_UAV_Task3/Position Controller/ADAPTIVE CONTROLLER/Subsystem2/MATLAB Function1 ==
  data: u input; phi_a output; phip input
function phi_a = fcn(u, phip)

phi_a = [u(1,1), u(2,1), u(3,1);
    phip(1,1), phip(1,2), phip(1,3);
    phip(2,1), phip(2,2), phip(2,3);
    phip(3,1), phip(3,2), phip(3,3)];

== matlab function Simplified_UAV_Task3/Position Controller/ADAPTIVE CONTROLLER/Subsystem2/MATLAB Function4 ==
  data: theta_a input; lambda output; thetap_hat output
function [lambda, thetap_hat] = fcn(theta_a)

lambda = theta_a(1);
thetap_hat = [theta_a(2) theta_a(3) theta_a(4)]';

== matlab function Simplified_UAV_Task3/Position Controller/ADAPTIVE CONTROLLER/Subsystem2/Projection operator ==
  data: f output; theta_a_hat input; y_proj output; y input; epsilon_PO parameter; theta_M parameter; ygrad output
function [f, y_proj, ygrad] = fcn(theta_a_hat, y, epsilon_PO, theta_M)

% 1
f_1 = ((1 + epsilon_PO(1))*theta_a_hat(1)^2 - theta_M(1)^2)/(epsilon_PO(1)*theta_M(1)^2);
grad_f_1 = 2*(1 + epsilon_PO(1))*theta_a_hat(1)/(epsilon_PO(1)*theta_M(1)^2);

if f_1>0 && y(1)*grad_f_1>0
    y_proj_1 = y(1) - f_1*(grad_f_1^2)/grad_f_1^2*y(1);
else
    y_proj_1 = y(1);
end

% 2
f_2 = ((2 + epsilon_PO(2))*theta_a_hat(2)^2 - theta_M(2)^2)/(epsilon_PO(2)*theta_M(2)^2);
grad_f_2 = 2*(2 + epsilon_PO(2))*theta_a_hat(2)/(epsilon_PO(2)*theta_M(2)^2);

if f_2>0 && y(2)*grad_f_2>0
    y_proj_2 = y(2) - f_2*(grad_f_2^2)/grad_f_2^2*y(2);
else
    y_proj_2 = y(2);
end

% 3
f_3 = ((3 + epsilon_PO(3))*theta_a_hat(3)^2 - theta_M(3)^2)/(epsilon_PO(3)*theta_M(3)^2);
grad_f_3 = 2*(3 + epsilon_PO(3))*theta_a_hat(3)/(epsilon_PO(3)*theta_M(3)^2);

if f_3>0 && y(3)*grad_f_3>0
    y_proj_3 = y(3) - f_3*(grad_f_3^2)/grad_f_3^2*y(3);
else
    y_proj_3 = y(3);
end

% 4
f_4 = ((4 + epsilon_PO(4))*theta_a_hat(4)^2 - theta_M(4)^2)/(epsilon_PO(4)*theta_M(4)^2);
grad_f_4 = 2*(4 + epsilon_PO(4))*theta_a_hat(4)/(epsilon_PO(4)*theta_M(4)^2);

if f_4>0 && y(4)*grad_f_4>0
    y_proj_4 = y(4) - f_4*(grad_f_4^2)/grad_f_4^2*y(4);
else
    y_proj_4 = y(4);
end

f = [f_1, f_2, f_3, f_4]';
y_proj = [y_proj_1, y_proj_2, y_proj_3, y_proj_4]';
grad_f = [grad_f_1, grad_f_2, grad_f_3, grad_f_4]';
ygrad = [y(1)*grad_f_1, y(2)*grad_f_2, y(3)*grad_f_3, y(4)*grad_f_4];

== matlab function Simplified_UAV_Task3/Position Controller/Adaptive Augmentation/Subsystem/Inverse ==
  data: u input; y output
function y = fcn(u)

Lambda = diag([u;u;u]);
y = inv(Lambda);

== matlab function Simplified_UAV_Task3/Classic Position Controller/Position feedforward ==
  data: e_pos input; y output; a_d input; v_d input; v input; v_c_dot2 input; UAV parameter; ctrl parameter; par parameter
function y = fcn(e_pos,a_d,v_d,v,v_c_dot2,UAV,ctrl,par)

g = par.g;
e3 = par.e_3;
m = UAV.m;
v_M = 10;

Kpos = ctrl.Kpos;

v_c_dot = - (eye(3)- diag(tanh( Kpos * e_pos/v_M).^2))*Kpos*(v-v_d) + a_d;

y = m*(v_c_dot2-g*e3);

== matlab function Simplified_UAV_Task3/Adaptive Augmentation/Subsystem/Inverse ==
  data: u input; y output
function y = fcn(u)

Lambda = diag([u;u;u]);
y = inv(Lambda);

== matlab function Simplified_UAV_Task3/Position Controller/Adaptive Augmentation/theta_a_hat dynamics/Projection operator/MATLAB Function ==
  data: theta input; y_proj output; theta_dot input; par parameter
function y_proj = proj(theta,theta_dot,par)

% I could get rid of the center by not feeding it to the function

Gamma = par.Gamma(1);
eps_proj = par.eps_proj;
theta_M = par.theta_M(1);
center = par.center(1);
theta = theta - center;

f = 1/(eps_proj*theta_M^2)*((1+eps_proj)*(theta')*theta-theta_M^2);
grad_f = 2/(eps_proj*theta_M^2)*(1+eps_proj)*theta;

if f>0 && all(theta_dot'*Gamma*grad_f>0)
    y_proj = Gamma*theta_dot - f*Gamma*(grad_f)*grad_f'/(grad_f'*Gamma*grad_f)*Gamma*theta_dot;
else
    y_proj = Gamma*theta_dot;
end

== matlab function Simplified_UAV_Task3/Position Controller/Adaptive Augmentation/theta_a_hat dynamics/Projection operator/MATLAB Function3 ==
  data: theta input; y_proj output; theta_dot input; par parameter
function y_proj = proj(theta,theta_dot,par)

% I could get rid of the center by not feeding it to the function

Gamma = par.Gamma(2);
eps_proj = par.eps_proj;
theta_M = par.theta_M(2);
center = par.center(2);
theta = theta - center;

f = 1/(eps_proj*theta_M^2)*((1+eps_proj)*(theta')*theta-theta_M^2);
grad_f = 2/(eps_proj*theta_M^2)*(1+eps_proj)*theta;

if f>0 && all(theta_dot'*Gamma*grad_f>0)
    y_proj = Gamma*theta_dot - f*Gamma*(grad_f)*grad_f'/(grad_f'*Gamma*grad_f)*Gamma*theta_dot;
else
    y_proj = Gamma*theta_dot;
end

== matlab function Simplified_UAV_Task3/Position Controller/Adaptive Augmentation/theta_a_hat dynamics/Projection operator/MATLAB Function4 ==
  data: theta input; y_proj output; theta_dot input; par parameter
function y_proj = proj(theta,theta_dot,par)

% I could get rid of the center by not feeding it to the function

Gamma = par.Gamma(3);
eps_proj = par.eps_proj;
theta_M = par.theta_M(3);
center = par.center(3);
theta = theta - center;

f = 1/(eps_proj*theta_M^2)*((1+eps_proj)*(theta')*theta-theta_M^2);
grad_f = 2/(eps_proj*theta_M^2)*(1+eps_proj)*theta;

if f>0 && all(theta_dot'*Gamma*grad_f>0)
    y_proj = Gamma*theta_dot - f*Gamma*(grad_f)*grad_f'/(grad_f'*Gamma*grad_f)*Gamma*theta_dot;
else
    y_proj = Gamma*theta_dot;
end

== matlab function Simplified_UAV_Task3/Position Controller/Adaptive Augmentation/theta_a_hat dynamics/Projection operator/MATLAB Function5 ==
  data: theta input; y_proj output; theta_dot input; par parameter
function y_proj = proj(theta,theta_dot,par)

% I could get rid of the center by not feeding it to the function

Gamma = par.Gamma(4);
eps_proj = par.eps_proj;
theta_M = par.theta_M(4);
center = par.center(4);
theta = theta - center;

f = 1/(eps_proj*theta_M^2)*((1+eps_proj)*(theta')*theta-theta_M^2);
grad_f = 2/(eps_proj*theta_M^2)*(1+eps_proj)*theta;

if f>0 && all(theta_dot'*Gamma*grad_f>0)
    y_proj = Gamma*theta_dot - f*Gamma*(grad_f)*grad_f'/(grad_f'*Gamma*grad_f)*Gamma*theta_dot;
else
    y_proj = Gamma*theta_dot;
end

== matlab function Simplified_UAV_Task3/Classic Position Controller/Adaptive Augmentation/Subsystem/Inverse ==
  data: u input; y output
function y = fcn(u)

Lambda = diag([u;u;u]);
y = inv(Lambda);

== matlab function Simplified_UAV_Task3/Classic Position Controller/Adaptive Augmentation/theta_a_hat dynamics/Projection operator/MATLAB Function ==
  data: theta input; y_proj output; theta_dot input; par parameter
function y_proj = proj(theta,theta_dot,par)

% I could get rid of the center by not feeding it to the function

Gamma = par.Gamma(1);
eps_proj = par.eps_proj;
theta_M = par.theta_M(1);
center = par.center(1);
theta = theta - center;

f = 1/(eps_proj*theta_M^2)*((1+eps_proj)*(theta')*theta-theta_M^2);
grad_f = 2/(eps_proj*theta_M^2)*(1+eps_proj)*theta;

if f>0 && all(theta_dot'*Gamma*grad_f>0)
    y_proj = Gamma*theta_dot - f*Gamma*(grad_f)*grad_f'/(grad_f'*Gamma*grad_f)*Gamma*theta_dot;
else
    y_proj = Gamma*theta_dot;
end

== matlab function Simplified_UAV_Task3/Classic Position Controller/Adaptive Augmentation/theta_a_hat dynamics/Projection operator/MATLAB Function3 ==
  data: theta input; y_proj output; theta_dot input; par parameter
function y_proj = proj(theta,theta_dot,par)

% I could get rid of the center by not feeding it to the function

Gamma = par.Gamma(2);
eps_proj = par.eps_proj;
theta_M = par.theta_M(2);
center = par.center(2);
theta = theta - center;

f = 1/(eps_proj*theta_M^2)*((1+eps_proj)*(theta')*theta-theta_M^2);
grad_f = 2/(eps_proj*theta_M^2)*(1+eps_proj)*theta;

if f>0 && all(theta_dot'*Gamma*grad_f>0)
    y_proj = Gamma*theta_dot - f*Gamma*(grad_f)*grad_f'/(grad_f'*Gamma*grad_f)*Gamma*theta_dot;
else
    y_proj = Gamma*theta_dot;
end

== matlab function Simplified_UAV_Task3/Classic Position Controller/Adaptive Augmentation/theta_a_hat dynamics/Projection operator/MATLAB Function4 ==
  data: theta input; y_proj output; theta_dot input; par parameter
function y_proj = proj(theta,theta_dot,par)

% I could get rid of the center by not feeding it to the function

Gamma = par.Gamma(3);
eps_proj = par.eps_proj;
theta_M = par.theta_M(3);
center = par.center(3);
theta = theta - center;

f = 1/(eps_proj*theta_M^2)*((1+eps_proj)*(theta')*theta-theta_M^2);
grad_f = 2/(eps_proj*theta_M^2)*(1+eps_proj)*theta;

if f>0 && all(theta_dot'*Gamma*grad_f>0)
    y_proj = Gamma*theta_dot - f*Gamma*(grad_f)*grad_f'/(grad_f'*Gamma*grad_f)*Gamma*theta_dot;
else
    y_proj = Gamma*theta_dot;
end

== matlab function Simplified_UAV_Task3/Adaptive Augmentation 6 parameters/Subsystem/Inverse ==
  data: u input; y output
function y = fcn(u)

y = inv(u);

== matlab function Simplified_UAV_Task3/Classic Position Controller/Adaptive Augmentation/theta_a_hat dynamics/Projection operator/MATLAB Function5 ==
  data: theta input; y_proj output; theta_dot input; par parameter
function y_proj = proj(theta,theta_dot,par)

% I could get rid of the center by not feeding it to the function

Gamma = par.Gamma(4);
eps_proj = par.eps_proj;
theta_M = par.theta_M(4);
center = par.center(4);
theta = theta - center;

f = 1/(eps_proj*theta_M^2)*((1+eps_proj)*(theta')*theta-theta_M^2);
grad_f = 2/(eps_proj*theta_M^2)*(1+eps_proj)*theta;

if f>0 && all(theta_dot'*Gamma*grad_f>0)
    y_proj = Gamma*theta_dot - f*Gamma*(grad_f)*grad_f'/(grad_f'*Gamma*grad_f)*Gamma*theta_dot;
else
    y_proj = Gamma*theta_dot;
end

== matlab function Simplified_UAV_Task3/Adaptive Augmentation 6 parameters/theta_a_hat dynamics/Projection operator/MATLAB Function ==
  data: theta input; y_proj output; theta_dot input; par parameter
function y_proj = proj(theta,theta_dot,par)

% I could get rid of the center by not feeding it to the function

Gamma = par.Gamma(1);
eps_proj = par.eps_proj;
theta_M = par.theta_M(1);
center = par.center(1);
theta = theta - center;

f = 1/(eps_proj*theta_M^2)*((1+eps_proj)*(theta')*theta-theta_M^2);
grad_f = 2/(eps_proj*theta_M^2)*(1+eps_proj)*theta;

if f>0 && all(theta_dot'*Gamma*grad_f>0)
    y_proj = Gamma*theta_dot - f*Gamma*(grad_f)*grad_f'/(grad_f'*Gamma*grad_f)*Gamma*theta_dot;
else
    y_proj = Gamma*theta_dot;
end

== matlab function Simplified_UAV_Task3/Adaptive Augmentation/theta_a_hat dynamics/Projection operator/MATLAB Function3 ==
  data: theta input; y_proj output; theta_dot input; par parameter
function y_proj = proj(theta,theta_dot,par)

% I could get rid of the center by not feeding it to the function

Gamma = par.Gamma(4);
eps_proj = par.eps_proj;
theta_M = par.theta_M(4);
center = par.center(4);
theta = theta - center;

f = 1/(eps_proj*theta_M^2)*((1+eps_proj)*(theta')*theta-theta_M^2);
grad_f = 2/(eps_proj*theta_M^2)*(1+eps_proj)*theta;

if f>0 && all(theta_dot'*Gamma*grad_f>0)
    y_proj = Gamma*theta_dot - f*Gamma*(grad_f)*grad_f'/(grad_f'*Gamma*grad_f)*Gamma*theta_dot;
else
    y_proj = Gamma*theta_dot;
end

== matlab function Simplified_UAV_Task3/Adaptive Augmentation/theta_a_hat dynamics/Projection operator/MATLAB Function4 ==
  data: theta input; y_proj output; theta_dot input; par parameter
function y_proj = proj(theta,theta_dot,par)

% I could get rid of the center by not feeding it to the function

Gamma = par.Gamma(5);
eps_proj = par.eps_proj;
theta_M = par.theta_M(5);
center = par.center(5);
theta = theta - center;

f = 1/(eps_proj*theta_M^2)*((1+eps_proj)*(theta')*theta-theta_M^2);
grad_f = 2/(eps_proj*theta_M^2)*(1+eps_proj)*theta;

if f>0 && all(theta_dot'*Gamma*grad_f>0)
    y_proj = Gamma*theta_dot - f*Gamma*(grad_f)*grad_f'/(grad_f'*Gamma*grad_f)*Gamma*theta_dot;
else
    y_proj = Gamma*theta_dot;
end

== matlab function Simplified_UAV_Task3/Adaptive Augmentation/theta_a_hat dynamics/Projection operator/MATLAB Function5 ==
  data: theta input; y_proj output; theta_dot input; par parameter
function y_proj = proj(theta,theta_dot,par)

% I could get rid of the center by not feeding it to the function

Gamma = par.Gamma(4);
eps_proj = par.eps_proj;
theta_M = par.theta_M(4);
center = par.center(4);
theta = theta - center;

f = 1/(eps_proj*theta_M^2)*((1+eps_proj)*(theta')*theta-theta_M^2);
grad_f = 2/(eps_proj*theta_M^2)*(1+eps_proj)*theta;

if f>0 && all(theta_dot'*Gamma*grad_f>0)
    y_proj = Gamma*theta_dot - f*Gamma*(grad_f)*grad_f'/(grad_f'*Gamma*grad_f)*Gamma*theta_dot;
else
    y_proj = Gamma*theta_dot;
end

== matlab function Simplified_UAV_Task3/ADAPTIVE CONTROLLER/Subsystem1/MATLAB Function1 ==
  data: lambda input; Lambda_hat_inv output
function Lambda_hat_inv = fcn(lambda)

%lambda_hat = [lambda 0 0; 0 lambda 0; 0 0 lambda];
Lambda_hat_inv = inv(lambda);

== matlab function Simplified_UAV_Task3/Adaptive Augmentation 6 parameters/theta_a_hat dynamics/Projection operator/MATLAB Function3 ==
  data: theta input; y_proj output; theta_dot input; par parameter
function y_proj = proj(theta,theta_dot,par)

% I could get rid of the center by not feeding it to the function

Gamma = par.Gamma(4);
eps_proj = par.eps_proj;
theta_M = par.theta_M(4);
center = par.center(4);
theta = theta - center;

f = 1/(eps_proj*theta_M^2)*((1+eps_proj)*(theta')*theta-theta_M^2);
grad_f = 2/(eps_proj*theta_M^2)*(1+eps_proj)*theta;

if f>0 && all(theta_dot'*Gamma*grad_f>0)
    y_proj = Gamma*theta_dot - f*Gamma*(grad_f)*grad_f'/(grad_f'*Gamma*grad_f)*Gamma*theta_dot;
else
    y_proj = Gamma*theta_dot;
end

== matlab function Simplified_UAV_Task3/Adaptive Augmentation 6 parameters/theta_a_hat dynamics/Projection operator/MATLAB Function4 ==
  data: theta input; y_proj output; theta_dot input; par parameter
function y_proj = proj(theta,theta_dot,par)

% I could get rid of the center by not feeding it to the function

Gamma = par.Gamma(5);
eps_proj = par.eps_proj;
theta_M = par.theta_M(5);
center = par.center(5);
theta = theta - center;

f = 1/(eps_proj*theta_M^2)*((1+eps_proj)*(theta')*theta-theta_M^2);
grad_f = 2/(eps_proj*theta_M^2)*(1+eps_proj)*theta;

if f>0 && all(theta_dot'*Gamma*grad_f>0)
    y_proj = Gamma*theta_dot - f*Gamma*(grad_f)*grad_f'/(grad_f'*Gamma*grad_f)*Gamma*theta_dot;
else
    y_proj = Gamma*theta_dot;
end
